simulink library "TCU_GS"  (R2025b)
settings: Solver=VariableStepAuto  StartTime=0.0  StopTime=10.0  RelTol=1e-3
settings Model: Creator=joshu  LastModifiedBy=joshu

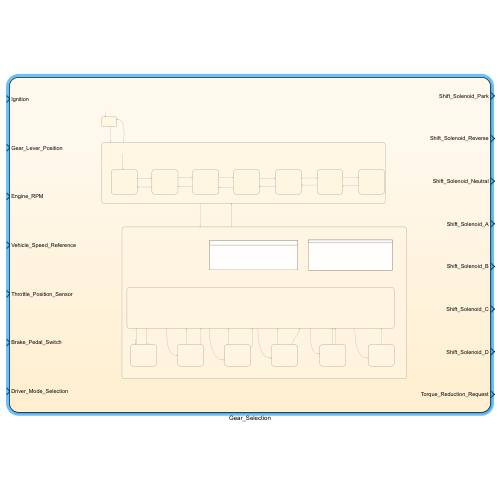
[thumbnail: Simulink's stored preview of the top-level diagram]
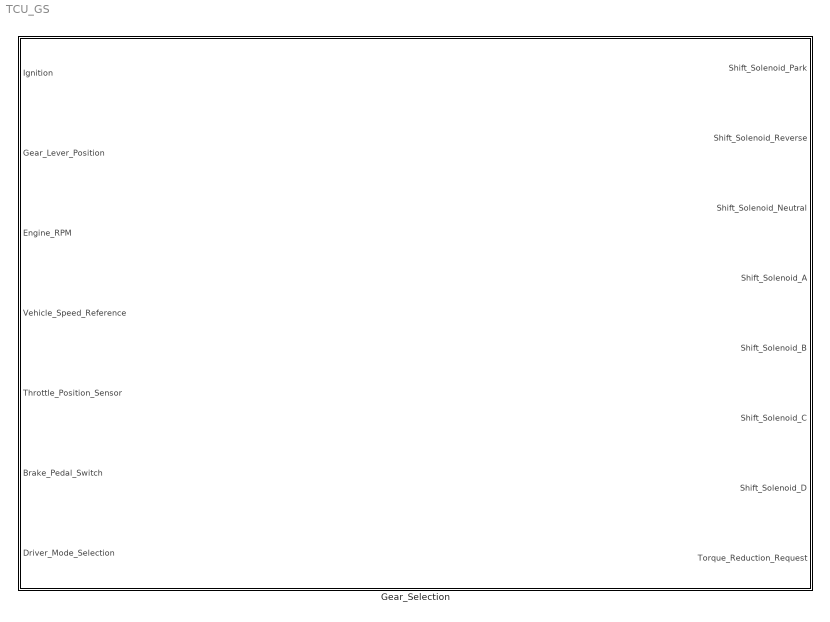
== system TCU_GS ==
  Gear_Selection : Stateflow chart  TreatAsAtomicUnit=on

== stateflow chart TCU_GS/Gear_Selection ==
  state Off
  state Selection
    state reverse
      during:
      Shift_Solenoid_Park=0;
      Shift_Solenoid_Reverse=1;
      Shift_Solenoid_Neutral=0;
      D=0;
    state neutral
      during:
      Shift_Solenoid_Park=0;
      Shift_Solenoid_Reverse=0;
      Shift_Solenoid_Neutral=1;
      D=0;
    state drive
      during:
      Shift_Solenoid_Park=0;
      Shift_Solenoid_Reverse=0;
      Shift_Solenoid_Neutral=0;
      D=1;
    state primera
      during:
      Shift_Solenoid_Park=0;
      Shift_Solenoid_Reverse=0;
      Shift_Solenoid_Neutral=0;
      D=1;
    state segunda
      during:
      Shift_Solenoid_Park=0;
      Shift_Solenoid_Reverse=0;
      Shift_Solenoid_Neutral=0;
      D=1;
    state tercera
      during:
      Shift_Solenoid_Park=0;
      Shift_Solenoid_Reverse=0;
      Shift_Solenoid_Neutral=0;
      D=1;
    state parking
      during:
      Shift_Solenoid_Park=1;
      Shift_Solenoid_Reverse=0;
      Shift_Solenoid_Neutral=0;
      D=0;
    (default) -> parking
    neutral -> drive [order 1] : [Gear_Lever_Position==4]
    segunda -> tercera [order 1] : [Gear_Lever_Position==32]
    reverse -> neutral [order 1] : [Gear_Lever_Position==2]
    primera -> segunda [order 1] : [Gear_Lever_Position==16]
    drive -> primera [order 1] : [Gear_Lever_Position==8]
    parking -> reverse : [Gear_Lever_Position==1 && Brake_Pedal_Switch == 1]
    segunda -> primera [order 2] : [Gear_Lever_Position==8]
    tercera -> segunda : [Gear_Lever_Position==16]
    primera -> drive [order 2] : [Gear_Lever_Position==4]
    neutral -> reverse [order 2] : [Gear_Lever_Position==1]
    reverse -> parking [order 2] : [Gear_Lever_Position==0 && Brake_Pedal_Switch == 1]
    drive -> neutral [order 2] : [Gear_Lever_Position==2]
  state Gear_Selection
    during:
    DriveStyle    = UpdateDriveStyle(Engine_RPM, Vehicle_Speed_Reference, Throttle_Position_Sensor);
    Objective_Gear = GearSelector(Engine_RPM, Vehicle_Speed_Reference, Throttle_Position_Sensor, Current_Gear_State, Driver_Mode_Selection, DriveStyle);
    state Shifting
      entry:
      Torque_Reduction_Request = 1;
      during:
      after(1,sec)
      Torque_Reduction_Request = 0;
    state First
      entry:
      Current_Gear_State = 1;
      during:
      Shift_Solenoid_A = 1;
      Shift_Solenoid_B = 0;
      Shift_Solenoid_C = 0;
      Shift_Solenoid_D = 0;
    state Second
      entry:
      Current_Gear_State = 2;
      during:
      Shift_Solenoid_A = 1;
      Shift_Solenoid_B = 1;
      Shift_Solenoid_C = 0;
      Shift_Solenoid_D = 0;
    state Third
      entry:
      Current_Gear_State = 3;
      during:
      Shift_Solenoid_A = 1;
      Shift_Solenoid_B = 1;
      Shift_Solenoid_C = 1;
      Shift_Solenoid_D = 0;
    state Fourth
      entry:
      Current_Gear_State = 4;
      during:
      Shift_Solenoid_A = 0;
      Shift_Solenoid_B = 1;
      Shift_Solenoid_C = 1;
      Shift_Solenoid_D = 0;
    state Fifth
      entry:
      Current_Gear_State = 5;
      during:
      Shift_Solenoid_A = 0;
      Shift_Solenoid_B = 0;
      Shift_Solenoid_C = 1;
      Shift_Solenoid_D = 1;
    state Sixth
      entry:
      Current_Gear_State = 6;
      during:
      Shift_Solenoid_A = 0;
      Shift_Solenoid_B = 0;
      Shift_Solenoid_C = 0;
      Shift_Solenoid_D = 1;
    First -> Shifting : [(Objective_Gear - Current_Gear_State)>0]
    Shifting -> First [order 1] : [Objective_Gear == 1 && Torque_Reduction_Request == 0]
    Shifting -> Second [order 2] : [Objective_Gear == 2 && Torque_Reduction_Request == 0]
    Second -> Shifting [order 1] : [(Objective_Gear-Current_Gear_State)<0]
    Second -> Shifting [order 2] : [(Objective_Gear-Current_Gear_State)>0]
    Shifting -> Third [order 3] : [Objective_Gear == 3 && Torque_Reduction_Request == 0]
    Third -> Shifting [order 2] : [(Objective_Gear-Current_Gear_State)<0]
    Third -> Shifting [order 1] : [(Objective_Gear-Current_Gear_State)>0]
    Shifting -> Fourth [order 4] : [Objective_Gear == 4 && Torque_Reduction_Request == 0]
    Fourth -> Shifting [order 2] : [(Objective_Gear-Current_Gear_State)<0]
    Fourth -> Shifting [order 1] : [(Objective_Gear-Current_Gear_State)>0]
    Shifting -> Fifth [order 5] : [Objective_Gear == 5 && Torque_Reduction_Request == 0]
    Fifth -> Shifting [order 2] : [(Objective_Gear-Current_Gear_State)<0]
    Fifth -> Shifting [order 1] : [(Objective_Gear-Current_Gear_State)>0]
    Shifting -> Sixth [order 6] : [Objective_Gear == 6 && Torque_Reduction_Request == 0]
    Sixth -> Shifting : [(Objective_Gear-Current_Gear_State)<0]
    (default) -> First
  (default) -> Off
  Selection -> Off [order 1] : [Ignition==0]
  Off -> Selection : [Ignition==2]
  Selection -> Gear_Selection [order 2] : [D == 1]
  Gear_Selection -> Selection : [D == 0]
  data: Engine_RPM function_input; VehSpeed_kph function_input; Throttle_pct function_input; DriveStyle function_output; Engine_RPM function_input; VehSpeed_kph function_input; Throttle_pct function_input; Actual_Gear function_input; DriveMode function_input; DriveStyle function_input; Objective_Gear function_output; Ignition input; Gear_Lever_Position input; Engine_RPM input; Vehicle_Speed_Reference input; Throttle_Position_Sensor input; Shift_Solenoid_Park output; Shift_Solenoid_Reverse output; Shift_Solenoid_Neutral output; Shift_Solenoid_A output; Shift_Solenoid_B output; Shift_Solenoid_C output; Shift_Solenoid_D output; Torque_Reduction_Request output; Brake_Pedal_Switch input; D local; Driver_Mode_Selection input; Current_Gear_State local; Objective_Gear local; DriveStyle local
  function DriveStyle = UpdateDriveStyle(Engine_RPM, VehSpeed_kph, Throttle_pct):
    | function DriveStyle = UpdateDriveStyle(Engine_RPM, VehSpeed_kph, Throttle_pct)
    | % UpdateDriveStyle
    | % Aprende un "estilo de manejo" adaptativo en rango [-1..+1]
    | %  -1  → manejo relajado
    | %  +1  → manejo agresivo
    | %
    | % Entradas:
    | %   Engine_RPM    : RPM motor
    | %   VehSpeed_kph  : Velocidad vehículo [km/h]
    | %   Throttle_pct  : Posición de acelerador [0..100]
    | %
    | % Salida:
    | %   DriveStyle    : Estilo de manejo [-1..+1] (promedio filtrado en el tiempo)
    | %
    | % NOTA: Pensado para llamarse periódicamente (ej. cada 50 ms)
    | 
    |     % ==== Persistentes (memoria entre llamadas) ====
    |     persistent styleState prevSpeed initialized
    |     
    |     if isempty(initialized)
    |         styleState  = 0;                % estilo inicial neutro
    |         prevSpeed   = VehSpeed_kph;     % para cálculo de aceleración
    |         initialized = true;
    |     end
    | 
    |     % ==== Parámetros de calibración ====
    |     % Tiempo de muestreo aproximado (segundos)
    |     Ts = 0.05;  % 50 ms, ajusta según tu sistema real
    | 
    |     % Rango de RPM en el que consideramos "uso fuerte"
    |     rpmLow  = 1500;
    |     rpmHigh = 3500;
    | 
    |     % Aceleración "alta" típica (para normalizar) [m/s^2]
    |     aHigh = 3.0;  % 0–3 m/s^2 rango relevante
    | 
    |     % Pesos de cada contribución a la agresividad instantánea
    |     wThrottle = 0.5;
    |     wRpm      = 0.3;
    |     wAccel    = 0.2;
    | 
    |     % Ganancia del filtro (qué tan rápido se adapta el estilo)
    |     % valor pequeño = aprendizaje más lento (más memoria)
    |     alpha = 0.02;     % 2% del error por llamada
    | 
    |     % ==== Sanitizar entradas ====
    |     Throttle_pct = max(0, min(100, Throttle_pct));
    |     Engine_RPM   = max(0, Engine_RPM);
    |     VehSpeed_kph = max(0, VehSpeed_kph);
    | 
    |     % ==== Cálculo de aceleración aproximada ====
    |     % v [km/h] → [m/s]: v_mps = v_kph / 3.6
    |     dv_kph     = VehSpeed_kph - prevSpeed;
    |     a_mps2     = (dv_kph / 3.6) / Ts;  % derivada simple
    |     prevSpeed  = VehSpeed_kph;        % actualizar memoria
    | 
    |     % Sólo usamos aceleración positiva para "agresividad"
    |     a_pos      = max(a_mps2, 0);
    |     accelNorm  = min(a_pos / aHigh, 1.0);  % 0..1
    | 
    |     % ==== Normalizar RPM y Throttle ====
    |     % Throttle 0–100 → 0..1
    |     thrNorm = Throttle_pct / 100;
    | 
    |     % RPM → 0..1 en [rpmLow, rpmHigh]
    |     rpmNorm = (Engine_RPM - rpmLow) / (rpmHigh - rpmLow);
    |     rpmNorm = max(0, min(1, rpmNorm));
    | 
    |     % ==== Métrica de agresividad instantánea (0..1) ====
    |     % 0  → muy relajado
    |     % 1  → muy agresivo
    |     aggressivenessInst = wThrottle * thrNorm + ...
    |                          wRpm      * rpmNorm + ...
    |                          wAccel    * accelNorm;
    | 
    |     % Asegurar rango 0..1
    |     aggressivenessInst = max(0, min(1, aggressivenessInst));
    | 
    |     % ==== Convertir a estilo [-1..+1] ====
    |     % 0.5 es un punto "neutro":
    |     %  >0.5 → positivo (agresivo), <0.5 → negativo (relajado)
    |     styleInst = 2 * (aggressivenessInst - 0.5);  % mapea 0..1 a -1..+1
    | 
    |     % ==== Filtro adaptativo (promedio exponencial) ====
    |     styleState = styleState + alpha * (styleInst - styleState);
    | 
    |     % ==== Saturación final y salida ====
    |     DriveStyle = max(-1, min(1, styleState));
    | 
    | end
  function Objective_Gear = GearSelector(Engine_RPM, VehSpeed_kph, Throttle_pct, ...:
    | function Objective_Gear = GearSelector(Engine_RPM, VehSpeed_kph, Throttle_pct, ...
    |                                        Actual_Gear, DriveMode, DriveStyle)
    | % GearSelector
    | %   Calcula la marcha objetivo en base a:
    | %   - RPM motor
    | %   - Velocidad vehículo [km/h]
    | %   - Posición de acelerador [%]
    | %   - Marcha actual
    | %   - Modo de manejo (0=Eco,1=Normal,2=Sport)
    | %   - Estilo de manejo [-1..+1] (relajado → -1, agresivo → +1)
    | 
    |     % ==== Calibraciones básicas ====
    |     MAX_GEAR = 6;
    |     MIN_GEAR = 1;
    |     
    |     % Umbrales base (modo NORMAL, throttle medio, estilo neutro)
    |     % Upshift: RPM para subir desde esa marcha a la siguiente
    |     %   1->2, 2->3, 3->4, 4->5, 5->6
    |     baseUpshiftRpm = [2200, 2400, 2600, 2600, 2600];  % [rpm]
    |     
    |     % Downshift: RPM por debajo de la cual se baja de marcha
    |     %   2->1, 3->2, 4->3, 5->4, 6->5
    |     baseDownshiftRpm = [1200, 1300, 1400, 1500, 1600]; % [rpm]
    |     
    |     % Factores por modo (escala RPM objetivo)
    |     %   Eco   → cambios más temprano (factor < 1)
    |     %   Normal→ factor 1
    |     %   Sport → cambios más tarde (factor > 1)
    |     modeFactorTable = [0.85, 1.0, 1.15];  % index: DriveMode+1
    |     
    |     % Influencia del estilo de manejo en los umbrales
    |     % DriveStyle = -1 → factor ≈ (1 - kStyle)
    |     % DriveStyle = +1 → factor ≈ (1 + kStyle)
    |     kStyle = 0.20;  % 20% de variación máxima por estilo
    |     
    |     % Influencia del acelerador (shift más tarde con más % pedal)
    |     kThrottleUp   = 4;   % rpm/%
    |     kThrottleDown = 2;   % rpm/% (menor influencia)
    |     
    |     % Kick-down
    |     kickdownThresh1 = 75;   % [%] primer nivel
    |     kickdownThresh2 = 90;   % [%] nivel fuerte
    |     kickdownMaxRpm  = 3500; % [rpm] por debajo de esto se permite bajar más
    |     
    |     % Protección básica por velocidad (muy simple, calibrable)
    |     minSpeedFor2 = 5;   % [km/h]
    |     minSpeedFor3 = 15;  % [km/h]
    |     minSpeedFor4 = 25;  % [km/h]
    |     minSpeedFor5 = 35;  % [km/h]
    |     minSpeedFor6 = 45;  % [km/h]
    |     minSpeedArray = [0, minSpeedFor2, minSpeedFor3, minSpeedFor4, ...
    |                         minSpeedFor5, minSpeedFor6]; % index por marcha
    |     
    |     % ==== Saturaciones básicas de entrada ====
    |     Throttle_pct = max(0, min(100, Throttle_pct));
    |     DriveStyle   = max(-1, min(1, DriveStyle));
    |     DriveMode    = max(0, min(2, DriveMode));
    |     Actual_Gear  = max(MIN_GEAR, min(MAX_GEAR, round(Actual_Gear)));
    |     
    |     % ==== Factores según modo y estilo ====
    |     modeFactor  = modeFactorTable(DriveMode + 1);
    |     styleFactor = 1 + kStyle * DriveStyle;
    |     
    |     % ==== Cálculo de umbrales para la marcha actual ====
    |     upRpm   = inf;
    |     downRpm = -inf;
    |     
    |     % Upshift (si no estamos ya en la última marcha)
    |     if Actual_Gear < MAX_GEAR
    |         idxUp = Actual_Gear; % 1->2 usa índice 1, etc.
    |         baseUp = baseUpshiftRpm(idxUp);
    |         upRpm = baseUp * modeFactor * styleFactor ...
    |                 + kThrottleUp * Throttle_pct;
    |     end
    |     
    |     % Downshift (si no estamos en la primera marcha)
    |     if Actual_Gear > MIN_GEAR
    |         idxDown = Actual_Gear - 1; % 2->1 usa índice 1, etc.
    |         baseDown = baseDownshiftRpm(idxDown);
    |         downRpm = baseDown * modeFactor * styleFactor ...
    |                   + kThrottleDown * Throttle_pct;
    |     end
    |     
    |     % ==== Lógica principal ====
    |     Objective_Gear = Actual_Gear;
    |     
    |     % 1) Protecciones por velocidad muy baja
    |     if VehSpeed_kph < 3
    |         Objective_Gear = 1;
    |         return;
    |     end
    |     
    |     % 2) Kick-down (prioridad sobre upshift)
    |     if Throttle_pct > kickdownThresh2 && Engine_RPM < kickdownMaxRpm
    |         % Kick-down fuerte: intentar bajar 2 marchas
    |         if Actual_Gear > (MIN_GEAR + 1)
    |             Objective_Gear = Actual_Gear - 2;
    |         elseif Actual_Gear > MIN_GEAR
    |             Objective_Gear = Actual_Gear - 1;
    |         end
    |         
    |     elseif Throttle_pct > kickdownThresh1 && Engine_RPM < (kickdownMaxRpm + 500)
    |         % Kick-down suave: bajar 1 marcha si se puede
    |         if Actual_Gear > MIN_GEAR
    |             Objective_Gear = Actual_Gear - 1;
    |         end
    |     else
    |         % 3) Lógica normal upshift/downshift
    |         %    (usamos primero downshift para mantener responsividad)
    |         
    |         % --- Downshift normal ---
    |         if (Engine_RPM < downRpm) && (Actual_Gear > MIN_GEAR)
    |             Objective_Gear = Actual_Gear - 1;
    |         end
    |         
    |         % --- Upshift normal ---
    |         % Solo si no cambiamos ya por downshift
    |         if Objective_Gear == Actual_Gear
    |             if (Engine_RPM > upRpm) && (Actual_Gear < MAX_GEAR)
    |                 % Además revisa velocidad mínima para la siguiente marcha
    |                 nextGear = Actual_Gear + 1;
    |                 if VehSpeed_kph >= minSpeedArray(nextGear)
    |                     Objective_Gear = nextGear;
    |                 end
    |             end
    |         end
    |     end
    |     
    |     % ==== Saturación final y chequeos ====
    |     Objective_Gear = max(MIN_GEAR, min(MAX_GEAR, Objective_Gear));
    |     
    |     % Seguridad extra: no permitir una marcha >1 si la velocidad
    |     % es inferior al mínimo calibrado de esa marcha.
    |     if VehSpeed_kph < minSpeedArray(Objective_Gear)
    |         % busca la marcha más alta permitida por velocidad
    |         allowedGear = MIN_GEAR;
    |         for g = MIN_GEAR:MAX_GEAR
    |             if VehSpeed_kph >= minSpeedArray(g)
    |                 allowedGear = g;
    |             else
    |                 break;
    |             end
    |         end
    |         Objective_Gear = allowedGear;
    |     end
    | 
    | end
